simulink model "Subsystem2"  (R2020a)
settings: Solver=VariableStepAuto  StartTime=0.0  StopTime=10.0  RelTol=1e-3
settings Model: Creator=tnradm  LastModifiedBy=tnradm
settings DataIOCC: SaveOutput=off  SaveTime=off

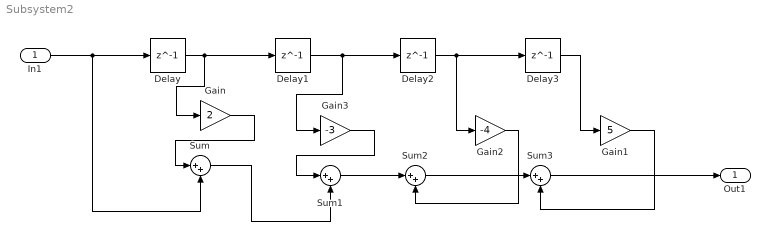
== system Subsystem2 ==
  In1 : Inport  OutDataTypeStr=double  PortDimensions=1  SampleTime=0
  Delay{,1..3} (4 alike) : Delay  DelayLength=1
  Gain : Gain  Gain=2
  Gain1 : Gain  Gain=5
  Gain2 : Gain  Gain=-4
  Gain3 : Gain  Gain=-3
  Sum{,1..3} (4 alike) : Sum  Inputs=|++
  Out1 : Outport  OutDataTypeStr=double  PortDimensions=1  SampleTime=0
  wires:
  Gain/1 -> Sum/1
  Gain3/1 -> Sum1/1
  Delay1/1 -> Gain3/1, Delay2/1
  In1/1 -> Delay/1, Sum/2
  Delay/1 -> Gain/1, Delay1/1
  Sum/1 -> Sum1/2
  Sum1/1 -> Sum2/1
  Delay2/1 -> Delay3/1, Gain2/1
  Sum2/1 -> Sum3/1
  Gain2/1 -> Sum2/2
  Gain1/1 -> Sum3/2
  Delay3/1 -> Gain1/1
  Sum3/1 -> Out1/1
